simulink library "halin"  (R2021b)
settings: Solver=VariableStepAuto  StartTime=0.0  StopTime=10.0  RelTol=1e-3
undefined symbols (not defined in the file): TRUE
libraries: FVT_lib x37, hcu_lib x31
(part 2 of 4)

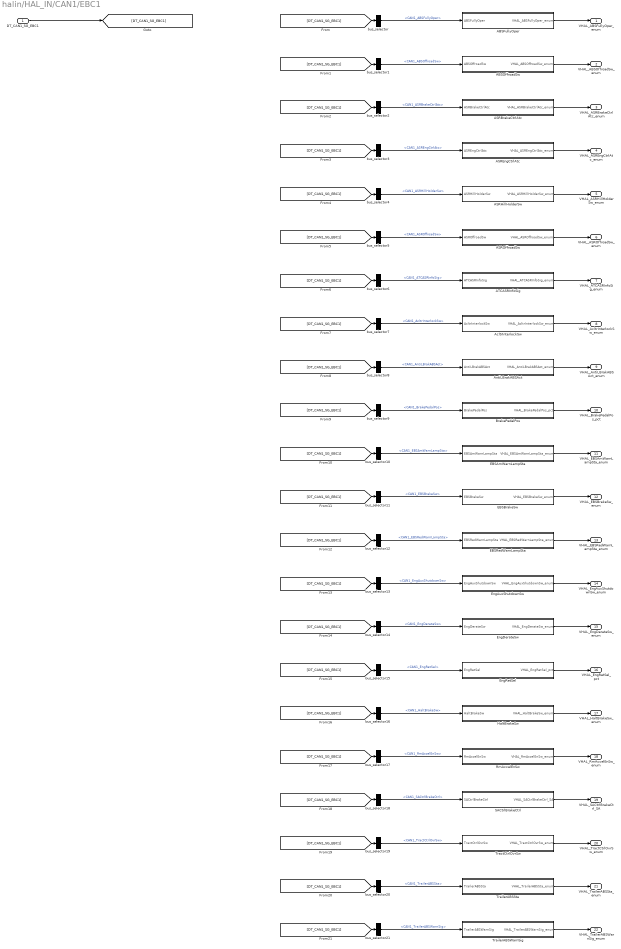
== system halin/HAL_IN/CAN1/EBC1 ==
  DT_CAN1_SG_EBC1 : Inport
  ABSFullyOper : Subsystem
  ABSOffroadSw : Subsystem
  ASRBrakeCtrlAtc : Subsystem
  ASREngCtrlAtc : Subsystem
  ASRHillHolderSw : Subsystem
  ASROffroadSw : Subsystem
  ATCASRInfoSig : Subsystem
  AcltrInterlockSw : Subsystem
  AntiLBrakABSAct : Subsystem
  BrakePedalPos : Subsystem
  EBSAmWarnLampSta : Subsystem
  EBSBrakeSw : Subsystem
  EBSRedWarnLampSta : Subsystem
  EngAuxShutdownSw : Subsystem
  EngDerateSw : Subsystem
  EngRetSel : Subsystem
  HaltBrakeSw : Subsystem
  RmAccelEnSw : Subsystem
  SACtrlBrakeCtrl : Subsystem
  TractCtrlOvrSw : Subsystem
  TrailerABSSta : Subsystem
  TrailerABSWarnSig : Subsystem
  bus_selector : BusSelector  OutputSignals=CAN1_ABSFullyOper
  bus_selector1 : BusSelector  OutputSignals=CAN1_ABSOffroadSw
  bus_selector10 : BusSelector  OutputSignals=CAN1_EBSAmWarnLampSta
  bus_selector11 : BusSelector  OutputSignals=CAN1_EBSBrakeSw
  bus_selector12 : BusSelector  OutputSignals=CAN1_EBSRedWarnLampSta
  bus_selector13 : BusSelector  OutputSignals=CAN1_EngAuxShutdownSw
  bus_selector14 : BusSelector  OutputSignals=CAN1_EngDerateSw
  bus_selector15 : BusSelector  OutputSignals=CAN1_EngRetSel
  bus_selector16 : BusSelector  OutputSignals=CAN1_HaltBrakeSw
  bus_selector17 : BusSelector  OutputSignals=CAN1_RmAccelEnSw
  bus_selector18 : BusSelector  OutputSignals=CAN1_SACtrlBrakeCtrl
  bus_selector19 : BusSelector  OutputSignals=CAN1_TractCtrlOvrSw
  bus_selector2 : BusSelector  OutputSignals=CAN1_ASRBrakeCtrlAtc
  bus_selector20 : BusSelector  OutputSignals=CAN1_TrailerABSSta
  bus_selector21 : BusSelector  OutputSignals=CAN1_TrailerABSWarnSig
  bus_selector3 : BusSelector  OutputSignals=CAN1_ASREngCtrlAtc
  bus_selector4 : BusSelector  OutputSignals=CAN1_ASRHillHolderSw
  bus_selector5 : BusSelector  OutputSignals=CAN1_ASROffroadSw
  bus_selector6 : BusSelector  OutputSignals=CAN1_ATCASRInfoSig
  bus_selector7 : BusSelector  OutputSignals=CAN1_AcltrInterlockSw
  bus_selector8 : BusSelector  OutputSignals=CAN1_AntiLBrakABSAct
  bus_selector9 : BusSelector  OutputSignals=CAN1_BrakePedalPos
  VHAL_ABSFullyOper_enum : Outport
  VHAL_ABSOffroadSw_enum : Outport  Port=2
  VHAL_ASRBrakeCtrlAtc_enum : Outport  Port=3
  VHAL_ASREngCtrlAtc_enum : Outport  Port=4
  VHAL_ASRHillHolderSw_enum : Outport  Port=5
  VHAL_ASROffroadSw_enum : Outport  Port=6
  VHAL_ATCASRInfoSig_enum : Outport  Port=7
  VHAL_AcltrInterlockSw_enum : Outport  Port=8
  VHAL_AntiLBrakABSAct_enum : Outport  Port=9
  VHAL_BrakePedalPos_pct : Outport  Port=10
  VHAL_EBSAmWarnLampSta_enum : Outport  Port=11
  VHAL_EBSBrakeSw_enum : Outport  Port=12
  VHAL_EBSRedWarnLampSta_enum : Outport  Port=13
  VHAL_EngAuxShutdownSw_enum : Outport  Port=14
  VHAL_EngDerateSw_enum : Outport  Port=15
  VHAL_EngRetSel_pct : Outport  Port=16
  VHAL_HaltBrakeSw_enum : Outport  Port=17
  VHAL_RmAccelEnSw_enum : Outport  Port=18
  VHAL_SACtrlBrakeCtrl_SA : Outport  Port=19
  VHAL_TractCtrlOvrSw_enum : Outport  Port=20
  VHAL_TrailerABSSta_enum : Outport  Port=21
  VHAL_TrailerABSWarnSig_enum : Outport  Port=22
  wires:
  DT_CAN1_SG_EBC1/1 -> [DT_CAN1_SG_EBC1]
  [DT_CAN1_SG_EBC1] -> bus_selector/1
  bus_selector/1 -> ABSFullyOper/1(ABSFullyOper)  "<CAN1_ABSFullyOper>"
  ABSFullyOper/1(VHAL_ABSFullyOper_enum) -> VHAL_ABSFullyOper_enum/1
  [DT_CAN1_SG_EBC1] -> bus_selector1/1
  bus_selector1/1 -> ABSOffroadSw/1(ABSOffroadSw)  "<CAN1_ABSOffroadSw>"
  ABSOffroadSw/1(VHAL_ABSOffroadSw_enum) -> VHAL_ABSOffroadSw_enum/1
  [DT_CAN1_SG_EBC1] -> bus_selector2/1
  bus_selector2/1 -> ASRBrakeCtrlAtc/1(ASRBrakeCtrlAtc)  "<CAN1_ASRBrakeCtrlAtc>"
  ASRBrakeCtrlAtc/1(VHAL_ASRBrakeCtrlAtc_enum) -> VHAL_ASRBrakeCtrlAtc_enum/1
  [DT_CAN1_SG_EBC1] -> bus_selector3/1
  bus_selector3/1 -> ASREngCtrlAtc/1(ASREngCtrlAtc)  "<CAN1_ASREngCtrlAtc>"
  ASREngCtrlAtc/1(VHAL_ASREngCtrlAtc_enum) -> VHAL_ASREngCtrlAtc_enum/1
  [DT_CAN1_SG_EBC1] -> bus_selector4/1
  bus_selector4/1 -> ASRHillHolderSw/1(ASRHillHolderSw)  "<CAN1_ASRHillHolderSw>"
  ASRHillHolderSw/1(VHAL_ASRHillHolderSw_enum) -> VHAL_ASRHillHolderSw_enum/1
  [DT_CAN1_SG_EBC1] -> bus_selector5/1
  bus_selector5/1 -> ASROffroadSw/1(ASROffroadSw)  "<CAN1_ASROffroadSw>"
  ASROffroadSw/1(VHAL_ASROffroadSw_enum) -> VHAL_ASROffroadSw_enum/1
  [DT_CAN1_SG_EBC1] -> bus_selector6/1
  bus_selector6/1 -> ATCASRInfoSig/1(ATCASRInfoSig)  "<CAN1_ATCASRInfoSig>"
  ATCASRInfoSig/1(VHAL_ATCASRInfoSig_enum) -> VHAL_ATCASRInfoSig_enum/1
  [DT_CAN1_SG_EBC1] -> bus_selector7/1
  bus_selector7/1 -> AcltrInterlockSw/1(AcltrInterlockSw)  "<CAN1_AcltrInterlockSw>"
  AcltrInterlockSw/1(VHAL_AcltrInterlockSw_enum) -> VHAL_AcltrInterlockSw_enum/1
  [DT_CAN1_SG_EBC1] -> bus_selector8/1
  bus_selector8/1 -> AntiLBrakABSAct/1(AntiLBrakABSAct)  "<CAN1_AntiLBrakABSAct>"
  AntiLBrakABSAct/1(VHAL_AntiLBrakABSAct_enum) -> VHAL_AntiLBrakABSAct_enum/1
  [DT_CAN1_SG_EBC1] -> bus_selector9/1
  bus_selector9/1 -> BrakePedalPos/1(BrakePedalPos)  "<CAN1_BrakePedalPos>"
  BrakePedalPos/1(VHAL_BrakePedalPos_pct) -> VHAL_BrakePedalPos_pct/1
  [DT_CAN1_SG_EBC1] -> bus_selector10/1
  bus_selector10/1 -> EBSAmWarnLampSta/1(EBSAmWarnLampSta)  "<CAN1_EBSAmWarnLampSta>"
  EBSAmWarnLampSta/1(VHAL_EBSAmWarnLampSta_enum) -> VHAL_EBSAmWarnLampSta_enum/1
  [DT_CAN1_SG_EBC1] -> bus_selector11/1
  bus_selector11/1 -> EBSBrakeSw/1(EBSBrakeSw)  "<CAN1_EBSBrakeSw>"
  EBSBrakeSw/1(VHAL_EBSBrakeSw_enum) -> VHAL_EBSBrakeSw_enum/1
  [DT_CAN1_SG_EBC1] -> bus_selector12/1
  bus_selector12/1 -> EBSRedWarnLampSta/1(EBSRedWarnLampSta)  "<CAN1_EBSRedWarnLampSta>"
  EBSRedWarnLampSta/1(VHAL_EBSRedWarnLampSta_enum) -> VHAL_EBSRedWarnLampSta_enum/1
  [DT_CAN1_SG_EBC1] -> bus_selector13/1
  bus_selector13/1 -> EngAuxShutdownSw/1(EngAuxShutdownSw)  "<CAN1_EngAuxShutdownSw>"
  EngAuxShutdownSw/1(VHAL_EngAuxShutdownSw_enum) -> VHAL_EngAuxShutdownSw_enum/1
  [DT_CAN1_SG_EBC1] -> bus_selector14/1
  bus_selector14/1 -> EngDerateSw/1(EngDerateSw)  "<CAN1_EngDerateSw>"
  EngDerateSw/1(VHAL_EngDerateSw_enum) -> VHAL_EngDerateSw_enum/1
  [DT_CAN1_SG_EBC1] -> bus_selector15/1
  bus_selector15/1 -> EngRetSel/1(EngRetSel)  "<CAN1_EngRetSel>"
  EngRetSel/1(VHAL_EngRetSel_pct) -> VHAL_EngRetSel_pct/1
  [DT_CAN1_SG_EBC1] -> bus_selector16/1
  bus_selector16/1 -> HaltBrakeSw/1(HaltBrakeSw)  "<CAN1_HaltBrakeSw>"
  HaltBrakeSw/1(VHAL_HaltBrakeSw_enum) -> VHAL_HaltBrakeSw_enum/1
  [DT_CAN1_SG_EBC1] -> bus_selector17/1
  bus_selector17/1 -> RmAccelEnSw/1(RmAccelEnSw)  "<CAN1_RmAccelEnSw>"
  RmAccelEnSw/1(VHAL_RmAccelEnSw_enum) -> VHAL_RmAccelEnSw_enum/1
  [DT_CAN1_SG_EBC1] -> bus_selector18/1
  bus_selector18/1 -> SACtrlBrakeCtrl/1(SACtrlBrakeCtrl)  "<CAN1_SACtrlBrakeCtrl>"
  SACtrlBrakeCtrl/1(VHAL_SACtrlBrakeCtrl_SA) -> VHAL_SACtrlBrakeCtrl_SA/1
  [DT_CAN1_SG_EBC1] -> bus_selector19/1
  bus_selector19/1 -> TractCtrlOvrSw/1(TractCtrlOvrSw)  "<CAN1_TractCtrlOvrSw>"
  TractCtrlOvrSw/1(VHAL_TractCtrlOvrSw_enum) -> VHAL_TractCtrlOvrSw_enum/1
  [DT_CAN1_SG_EBC1] -> bus_selector20/1
  bus_selector20/1 -> TrailerABSSta/1(TrailerABSSta)  "<CAN1_TrailerABSSta>"
  TrailerABSSta/1(VHAL_TrailerABSSta_enum) -> VHAL_TrailerABSSta_enum/1
  [DT_CAN1_SG_EBC1] -> bus_selector21/1
  bus_selector21/1 -> TrailerABSWarnSig/1(TrailerABSWarnSig)  "<CAN1_TrailerABSWarnSig>"
  TrailerABSWarnSig/1(VHAL_TrailerABSWarnSig_enum) -> VHAL_TrailerABSWarnSig_enum/1

== system halin/HAL_IN/CAN1/EBC2 ==
  DT_CAN1_SG_EBC2 : Inport
  FASpeed : Subsystem
  RelaSpdFALWheel : Subsystem
  RelaSpdFARWheel : Subsystem
  bus_selector : BusSelector  OutputSignals=CAN1_FASpeed
  bus_selector1 : BusSelector  OutputSignals=CAN1_RelaSpdFALWheel
  bus_selector2 : BusSelector  OutputSignals=CAN1_RelaSpdFARWheel
  VHAL_FASpeed_kph : Outport
  VHAL_RelaSpdFALWheel_kph : Outport  Port=2
  VHAL_RelaSpdFARWheel_kph : Outport  Port=3
  wires:
  DT_CAN1_SG_EBC2/1 -> [DT_CAN1_SG_EBC2]
  [DT_CAN1_SG_EBC2] -> bus_selector/1
  bus_selector/1 -> FASpeed/1(FASpeed)  "<CAN1_FASpeed>"
  FASpeed/1(VHAL_FASpeed_kph) -> VHAL_FASpeed_kph/1
  [DT_CAN1_SG_EBC2] -> bus_selector1/1
  bus_selector1/1 -> RelaSpdFALWheel/1(RelaSpdFALWheel)  "<CAN1_RelaSpdFALWheel>"
  RelaSpdFALWheel/1(VHAL_RelaSpdFALWheel_kph) -> VHAL_RelaSpdFALWheel_kph/1
  [DT_CAN1_SG_EBC2] -> bus_selector2/1
  bus_selector2/1 -> RelaSpdFARWheel/1(RelaSpdFARWheel)  "<CAN1_RelaSpdFARWheel>"
  RelaSpdFARWheel/1(VHAL_RelaSpdFARWheel_kph) -> VHAL_RelaSpdFARWheel_kph/1

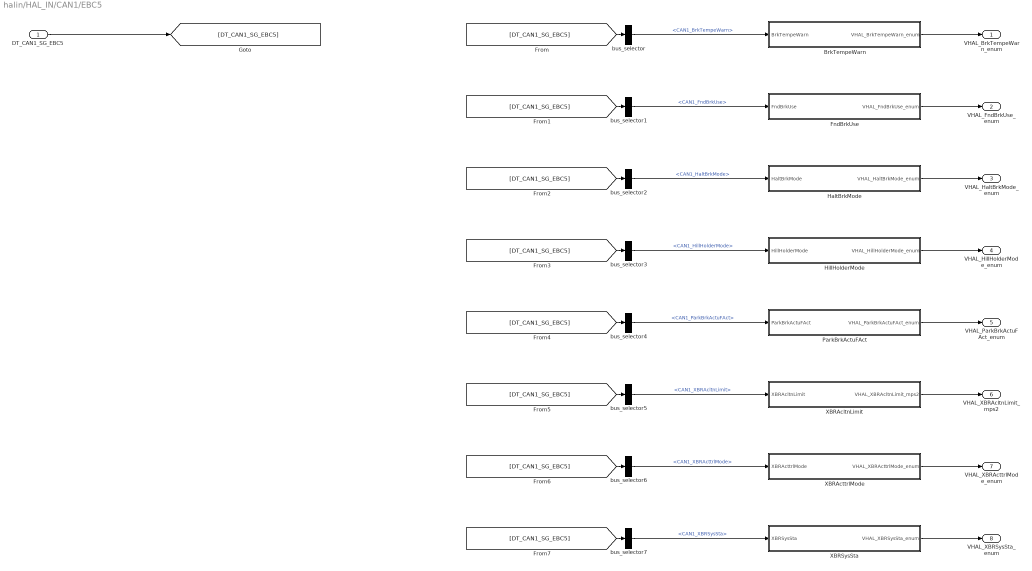
== system halin/HAL_IN/CAN1/EBC5 ==
  DT_CAN1_SG_EBC5 : Inport
  BrkTempeWarn : Subsystem
  FndBrkUse : Subsystem
  HaltBrkMode : Subsystem
  HillHolderMode : Subsystem
  ParkBrkActuFAct : Subsystem
  XBRAcltnLimit : Subsystem
  XBRActtrlMode : Subsystem
  XBRSysSta : Subsystem
  bus_selector : BusSelector  OutputSignals=CAN1_BrkTempeWarn
  bus_selector1 : BusSelector  OutputSignals=CAN1_FndBrkUse
  bus_selector2 : BusSelector  OutputSignals=CAN1_HaltBrkMode
  bus_selector3 : BusSelector  OutputSignals=CAN1_HillHolderMode
  bus_selector4 : BusSelector  OutputSignals=CAN1_ParkBrkActuFAct
  bus_selector5 : BusSelector  OutputSignals=CAN1_XBRAcltnLimit
  bus_selector6 : BusSelector  OutputSignals=CAN1_XBRActtrlMode
  bus_selector7 : BusSelector  OutputSignals=CAN1_XBRSysSta
  VHAL_BrkTempeWarn_enum : Outport
  VHAL_FndBrkUse_enum : Outport  Port=2
  VHAL_HaltBrkMode_enum : Outport  Port=3
  VHAL_HillHolderMode_enum : Outport  Port=4
  VHAL_ParkBrkActuFAct_enum : Outport  Port=5
  VHAL_XBRAcltnLimit_mps2 : Outport  Port=6
  VHAL_XBRActtrlMode_enum : Outport  Port=7
  VHAL_XBRSysSta_enum : Outport  Port=8
  wires:
  DT_CAN1_SG_EBC5/1 -> [DT_CAN1_SG_EBC5]
  [DT_CAN1_SG_EBC5] -> bus_selector/1
  bus_selector/1 -> BrkTempeWarn/1(BrkTempeWarn)  "<CAN1_BrkTempeWarn>"
  BrkTempeWarn/1(VHAL_BrkTempeWarn_enum) -> VHAL_BrkTempeWarn_enum/1
  [DT_CAN1_SG_EBC5] -> bus_selector1/1
  bus_selector1/1 -> FndBrkUse/1(FndBrkUse)  "<CAN1_FndBrkUse>"
  FndBrkUse/1(VHAL_FndBrkUse_enum) -> VHAL_FndBrkUse_enum/1
  [DT_CAN1_SG_EBC5] -> bus_selector2/1
  bus_selector2/1 -> HaltBrkMode/1(HaltBrkMode)  "<CAN1_HaltBrkMode>"
  HaltBrkMode/1(VHAL_HaltBrkMode_enum) -> VHAL_HaltBrkMode_enum/1
  [DT_CAN1_SG_EBC5] -> bus_selector3/1
  bus_selector3/1 -> HillHolderMode/1(HillHolderMode)  "<CAN1_HillHolderMode>"
  HillHolderMode/1(VHAL_HillHolderMode_enum) -> VHAL_HillHolderMode_enum/1
  [DT_CAN1_SG_EBC5] -> bus_selector4/1
  bus_selector4/1 -> ParkBrkActuFAct/1(ParkBrkActuFAct)  "<CAN1_ParkBrkActuFAct>"
  ParkBrkActuFAct/1(VHAL_ParkBrkActuFAct_enum) -> VHAL_ParkBrkActuFAct_enum/1
  [DT_CAN1_SG_EBC5] -> bus_selector5/1
  bus_selector5/1 -> XBRAcltnLimit/1(XBRAcltnLimit)  "<CAN1_XBRAcltnLimit>"
  XBRAcltnLimit/1(VHAL_XBRAcltnLimit_mps2) -> VHAL_XBRAcltnLimit_mps2/1
  [DT_CAN1_SG_EBC5] -> bus_selector6/1
  bus_selector6/1 -> XBRActtrlMode/1(XBRActtrlMode)  "<CAN1_XBRActtrlMode>"
  XBRActtrlMode/1(VHAL_XBRActtrlMode_enum) -> VHAL_XBRActtrlMode_enum/1
  [DT_CAN1_SG_EBC5] -> bus_selector7/1
  bus_selector7/1 -> XBRSysSta/1(XBRSysSta)  "<CAN1_XBRSysSta>"
  XBRSysSta/1(VHAL_XBRSysSta_enum) -> VHAL_XBRSysSta_enum/1

== system halin/HAL_IN/CAN1/ECAS_DM1 ==
  DT_CAN1_SG_ECAS_DM1 : Inport
  ECASAWarmLampSta : Subsystem
  bus_selector : BusSelector  OutputSignals=CAN1_ECASAWarmLampSta
  VHAL_ECASAWarmLampSta_enum : Outport
  wires:
  DT_CAN1_SG_ECAS_DM1/1 -> [DT_CAN1_SG_ECAS_DM1]
  [DT_CAN1_SG_ECAS_DM1] -> bus_selector/1
  bus_selector/1 -> ECASAWarmLampSta/1(ECASAWarmLampSta)  "<CAN1_ECASAWarmLampSta>"
  ECASAWarmLampSta/1(VHAL_ECASAWarmLampSta_enum) -> VHAL_ECASAWarmLampSta_enum/1

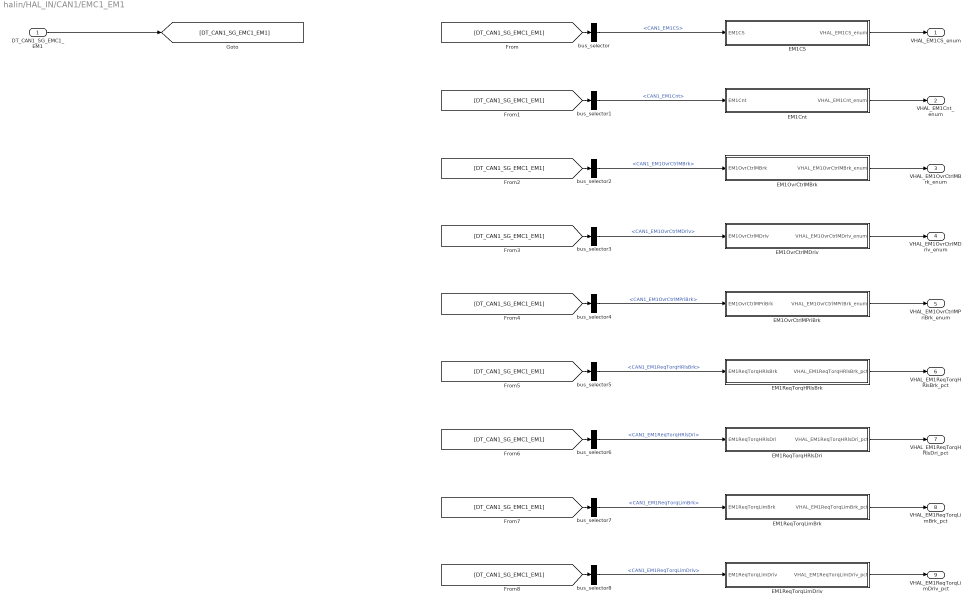
== system halin/HAL_IN/CAN1/EMC1_EM1 ==
  DT_CAN1_SG_EMC1_EM1 : Inport
  EM1CS : Subsystem
  EM1Cnt : Subsystem
  EM1OvrCtrlMBrk : Subsystem
  EM1OvrCtrlMDriv : Subsystem
  EM1OvrCtrlMPriBrk : Subsystem
  EM1ReqTorqHRlsBrk : Subsystem
  EM1ReqTorqHRlsDri : Subsystem
  EM1ReqTorqLimBrk : Subsystem
  EM1ReqTorqLimDriv : Subsystem
  bus_selector : BusSelector  OutputSignals=CAN1_EM1CS
  bus_selector1 : BusSelector  OutputSignals=CAN1_EM1Cnt
  bus_selector2 : BusSelector  OutputSignals=CAN1_EM1OvrCtrlMBrk
  bus_selector3 : BusSelector  OutputSignals=CAN1_EM1OvrCtrlMDriv
  bus_selector4 : BusSelector  OutputSignals=CAN1_EM1OvrCtrlMPriBrk
  bus_selector5 : BusSelector  OutputSignals=CAN1_EM1ReqTorqHRlsBrk
  bus_selector6 : BusSelector  OutputSignals=CAN1_EM1ReqTorqHRlsDri
  bus_selector7 : BusSelector  OutputSignals=CAN1_EM1ReqTorqLimBrk
  bus_selector8 : BusSelector  OutputSignals=CAN1_EM1ReqTorqLimDriv
  VHAL_EM1CS_enum : Outport
  VHAL_EM1Cnt_enum : Outport  Port=2
  VHAL_EM1OvrCtrlMBrk_enum : Outport  Port=3
  VHAL_EM1OvrCtrlMDriv_enum : Outport  Port=4
  VHAL_EM1OvrCtrlMPriBrk_enum : Outport  Port=5
  VHAL_EM1ReqTorqHRlsBrk_pct : Outport  Port=6
  VHAL_EM1ReqTorqHRlsDri_pct : Outport  Port=7
  VHAL_EM1ReqTorqLimBrk_pct : Outport  Port=8
  VHAL_EM1ReqTorqLimDriv_pct : Outport  Port=9
  wires:
  DT_CAN1_SG_EMC1_EM1/1 -> [DT_CAN1_SG_EMC1_EM1]
  [DT_CAN1_SG_EMC1_EM1] -> bus_selector/1
  bus_selector/1 -> EM1CS/1(EM1CS)  "<CAN1_EM1CS>"
  EM1CS/1(VHAL_EM1CS_enum) -> VHAL_EM1CS_enum/1
  [DT_CAN1_SG_EMC1_EM1] -> bus_selector1/1
  bus_selector1/1 -> EM1Cnt/1(EM1Cnt)  "<CAN1_EM1Cnt>"
  EM1Cnt/1(VHAL_EM1Cnt_enum) -> VHAL_EM1Cnt_enum/1
  [DT_CAN1_SG_EMC1_EM1] -> bus_selector2/1
  bus_selector2/1 -> EM1OvrCtrlMBrk/1(EM1OvrCtrlMBrk)  "<CAN1_EM1OvrCtrlMBrk>"
  EM1OvrCtrlMBrk/1(VHAL_EM1OvrCtrlMBrk_enum) -> VHAL_EM1OvrCtrlMBrk_enum/1
  [DT_CAN1_SG_EMC1_EM1] -> bus_selector3/1
  bus_selector3/1 -> EM1OvrCtrlMDriv/1(EM1OvrCtrlMDriv)  "<CAN1_EM1OvrCtrlMDriv>"
  EM1OvrCtrlMDriv/1(VHAL_EM1OvrCtrlMDriv_enum) -> VHAL_EM1OvrCtrlMDriv_enum/1
  [DT_CAN1_SG_EMC1_EM1] -> bus_selector4/1
  bus_selector4/1 -> EM1OvrCtrlMPriBrk/1(EM1OvrCtrlMPriBrk)  "<CAN1_EM1OvrCtrlMPriBrk>"
  EM1OvrCtrlMPriBrk/1(VHAL_EM1OvrCtrlMPriBrk_enum) -> VHAL_EM1OvrCtrlMPriBrk_enum/1
  [DT_CAN1_SG_EMC1_EM1] -> bus_selector5/1
  bus_selector5/1 -> EM1ReqTorqHRlsBrk/1(EM1ReqTorqHRlsBrk)  "<CAN1_EM1ReqTorqHRlsBrk>"
  EM1ReqTorqHRlsBrk/1(VHAL_EM1ReqTorqHRlsBrk_pct) -> VHAL_EM1ReqTorqHRlsBrk_pct/1
  [DT_CAN1_SG_EMC1_EM1] -> bus_selector6/1
  bus_selector6/1 -> EM1ReqTorqHRlsDri/1(EM1ReqTorqHRlsDri)  "<CAN1_EM1ReqTorqHRlsDri>"
  EM1ReqTorqHRlsDri/1(VHAL_EM1ReqTorqHRlsDri_pct) -> VHAL_EM1ReqTorqHRlsDri_pct/1
  [DT_CAN1_SG_EMC1_EM1] -> bus_selector7/1
  bus_selector7/1 -> EM1ReqTorqLimBrk/1(EM1ReqTorqLimBrk)  "<CAN1_EM1ReqTorqLimBrk>"
  EM1ReqTorqLimBrk/1(VHAL_EM1ReqTorqLimBrk_pct) -> VHAL_EM1ReqTorqLimBrk_pct/1
  [DT_CAN1_SG_EMC1_EM1] -> bus_selector8/1
  bus_selector8/1 -> EM1ReqTorqLimDriv/1(EM1ReqTorqLimDriv)  "<CAN1_EM1ReqTorqLimDriv>"
  EM1ReqTorqLimDriv/1(VHAL_EM1ReqTorqLimDriv_pct) -> VHAL_EM1ReqTorqLimDriv_pct/1

== system halin/HAL_IN/CAN1/HRW ==
  DT_CAN1_SG_HRW : Inport
  WhlSpeedFL : Subsystem
  bus_selector : BusSelector  OutputSignals=CAN1_WhlSpeed_FL
  VHAL_WhlSpeedFL_kph : Outport
  wires:
  DT_CAN1_SG_HRW/1 -> [DT_CAN1_SG_HRW]
  [DT_CAN1_SG_HRW] -> bus_selector/1
  bus_selector/1 -> WhlSpeedFL/1(WhlSpeed_FL)  "<CAN1_WhlSpeed_FL>"
  WhlSpeedFL/1(VHAL_WhlSpeedFL_kph) -> VHAL_WhlSpeedFL_kph/1

== system halin/HAL_IN/CAN1/TC1 ==
  DT_CAN1_SG_TC1 : Inport
  DrivDirF : Subsystem
  TransReqGear : Subsystem
  bus_selector : BusSelector  OutputSignals=CAN1_DrivDirF
  bus_selector1 : BusSelector  OutputSignals=CAN1_TransReqGear
  VHAL_DrivDirF_enum : Outport
  VHAL_TransReqGear_enum : Outport  Port=2
  wires:
  DT_CAN1_SG_TC1/1 -> [DT_CAN1_SG_TC1]
  [DT_CAN1_SG_TC1] -> bus_selector/1
  bus_selector/1 -> DrivDirF/1(DrivDirF)  "<CAN1_DrivDirF>"
  DrivDirF/1(VHAL_DrivDirF_enum) -> VHAL_DrivDirF_enum/1
  [DT_CAN1_SG_TC1] -> bus_selector1/1
  bus_selector1/1 -> TransReqGear/1(TransReqGear)  "<CAN1_TransReqGear>"
  TransReqGear/1(VHAL_TransReqGear_enum) -> VHAL_TransReqGear_enum/1

== system halin/HAL_IN/CAN1/VHAL_CANMsgInvalidACBTMSC10000_flg ==
  Cast To Boolean13 : DataTypeConversion  OutDataTypeStr=boolean
  Constant : Constant  Value=TRUE
  Latch13 : hcu_lib/Basic_Blocks/Latch
  Switch13 : Switch  Criteria=u2 ~= 0
  Unit Delay : UnitDelay  SampleTime=-1  HasFrameUpgradeWarning=on
  UnitConverter : DataTypeConversion  OutDataTypeStr=boolean
  Out : Outport
  wires:
  Constant/1 -> Switch13/3
  Unit Delay/1 -> Cast To Boolean13/1
  Cast To Boolean13/1 -> Switch13/1, Latch13/1
  Switch13/1 -> UnitConverter/1
  Latch13/1 -> Switch13/2
  UnitConverter/1 -> Unit Delay/1, Out/1  "VHAL_CANMsgInvalidACBTMSC10000_flg"

== system halin/HAL_IN/CAN1/VHAL_CANMsgInvalidACBTMSC10001_flg ==
  Cast To Boolean13 : DataTypeConversion  OutDataTypeStr=boolean
  Constant : Constant  Value=TRUE
  Latch13 : hcu_lib/Basic_Blocks/Latch
  Switch13 : Switch  Criteria=u2 ~= 0
  Unit Delay : UnitDelay  SampleTime=-1  HasFrameUpgradeWarning=on
  UnitConverter : DataTypeConversion  OutDataTypeStr=boolean
  Out : Outport
  wires:
  Constant/1 -> Switch13/3
  Unit Delay/1 -> Cast To Boolean13/1
  Cast To Boolean13/1 -> Switch13/1, Latch13/1
  Switch13/1 -> UnitConverter/1
  Latch13/1 -> Switch13/2
  UnitConverter/1 -> Unit Delay/1, Out/1  "VHAL_CANMsgInvalidACBTMSC10001_flg"

== system halin/HAL_IN/CAN1/VHAL_CANMsgInvalidACBTMSC10004_flg ==
  Cast To Boolean13 : DataTypeConversion  OutDataTypeStr=boolean
  Constant : Constant  Value=TRUE
  Latch13 : hcu_lib/Basic_Blocks/Latch
  Switch13 : Switch  Criteria=u2 ~= 0
  Unit Delay : UnitDelay  SampleTime=-1  HasFrameUpgradeWarning=on
  UnitConverter : DataTypeConversion  OutDataTypeStr=boolean
  Out : Outport
  wires:
  Constant/1 -> Switch13/3
  Unit Delay/1 -> Cast To Boolean13/1
  Cast To Boolean13/1 -> Switch13/1, Latch13/1
  Switch13/1 -> UnitConverter/1
  Latch13/1 -> Switch13/2
  UnitConverter/1 -> Unit Delay/1, Out/1  "VHAL_CANMsgInvalidACBTMSC10004_flg"

== system halin/HAL_IN/CAN1/VHAL_CANMsgInvalidACBTMSC50000_flg ==
  Cast To Boolean13 : DataTypeConversion  OutDataTypeStr=boolean
  Constant : Constant  Value=TRUE
  Latch13 : hcu_lib/Basic_Blocks/Latch
  Switch13 : Switch  Criteria=u2 ~= 0
  Unit Delay : UnitDelay  SampleTime=-1  HasFrameUpgradeWarning=on
  UnitConverter : DataTypeConversion  OutDataTypeStr=boolean
  Out : Outport
  wires:
  Constant/1 -> Switch13/3
  Unit Delay/1 -> Cast To Boolean13/1
  Cast To Boolean13/1 -> Switch13/1, Latch13/1
  Switch13/1 -> UnitConverter/1
  Latch13/1 -> Switch13/2
  UnitConverter/1 -> Unit Delay/1, Out/1  "VHAL_CANMsgInvalidACBTMSC50000_flg"

== system halin/HAL_IN/CAN1/VHAL_CANMsgInvalidASC1A_flg ==
  Cast To Boolean13 : DataTypeConversion  OutDataTypeStr=boolean
  Constant : Constant  Value=TRUE
  Latch13 : hcu_lib/Basic_Blocks/Latch
  Switch13 : Switch  Criteria=u2 ~= 0
  Unit Delay : UnitDelay  SampleTime=-1  HasFrameUpgradeWarning=on
  UnitConverter : DataTypeConversion  OutDataTypeStr=boolean
  Out : Outport
  wires:
  Constant/1 -> Switch13/3
  Unit Delay/1 -> Cast To Boolean13/1
  Cast To Boolean13/1 -> Switch13/1, Latch13/1
  Switch13/1 -> UnitConverter/1
  Latch13/1 -> Switch13/2
  UnitConverter/1 -> Unit Delay/1, Out/1  "VHAL_CANMsgInvalidASC1A_flg"

== system halin/HAL_IN/CAN1/VHAL_CANMsgInvalidEBC1_flg ==
  Cast To Boolean13 : DataTypeConversion  OutDataTypeStr=boolean
  Constant : Constant  Value=TRUE
  Latch13 : hcu_lib/Basic_Blocks/Latch
  Switch13 : Switch  Criteria=u2 ~= 0
  Unit Delay : UnitDelay  SampleTime=-1  HasFrameUpgradeWarning=on
  UnitConverter : DataTypeConversion  OutDataTypeStr=boolean
  Out : Outport
  wires:
  Constant/1 -> Switch13/3
  Unit Delay/1 -> Cast To Boolean13/1
  Cast To Boolean13/1 -> Switch13/1, Latch13/1
  Switch13/1 -> UnitConverter/1
  Latch13/1 -> Switch13/2
  UnitConverter/1 -> Unit Delay/1, Out/1  "VHAL_CANMsgInvalidEBC1_flg"

== system halin/HAL_IN/CAN1/VHAL_CANMsgInvalidEBC2_flg ==
  Cast To Boolean13 : DataTypeConversion  OutDataTypeStr=boolean
  Constant : Constant  Value=TRUE
  Latch13 : hcu_lib/Basic_Blocks/Latch
  Switch13 : Switch  Criteria=u2 ~= 0
  Unit Delay : UnitDelay  SampleTime=-1  HasFrameUpgradeWarning=on
  UnitConverter : DataTypeConversion  OutDataTypeStr=boolean
  Out : Outport
  wires:
  Constant/1 -> Switch13/3
  Unit Delay/1 -> Cast To Boolean13/1
  Cast To Boolean13/1 -> Switch13/1, Latch13/1
  Switch13/1 -> UnitConverter/1
  Latch13/1 -> Switch13/2
  UnitConverter/1 -> Unit Delay/1, Out/1  "VHAL_CANMsgInvalidEBC2_flg"

== system halin/HAL_IN/CAN1/VHAL_CANMsgInvalidEBC5_flg ==
  Cast To Boolean13 : DataTypeConversion  OutDataTypeStr=boolean
  Constant : Constant  Value=TRUE
  Latch13 : hcu_lib/Basic_Blocks/Latch
  Switch13 : Switch  Criteria=u2 ~= 0
  Unit Delay : UnitDelay  SampleTime=-1  HasFrameUpgradeWarning=on
  UnitConverter : DataTypeConversion  OutDataTypeStr=boolean
  Out : Outport
  wires:
  Constant/1 -> Switch13/3
  Unit Delay/1 -> Cast To Boolean13/1
  Cast To Boolean13/1 -> Switch13/1, Latch13/1
  Switch13/1 -> UnitConverter/1
  Latch13/1 -> Switch13/2
  UnitConverter/1 -> Unit Delay/1, Out/1  "VHAL_CANMsgInvalidEBC5_flg"

== system halin/HAL_IN/CAN1/VHAL_CANMsgInvalidECASDM1_flg ==
  Cast To Boolean13 : DataTypeConversion  OutDataTypeStr=boolean
  Constant : Constant  Value=TRUE
  Latch13 : hcu_lib/Basic_Blocks/Latch
  Switch13 : Switch  Criteria=u2 ~= 0
  Unit Delay : UnitDelay  SampleTime=-1  HasFrameUpgradeWarning=on
  UnitConverter : DataTypeConversion  OutDataTypeStr=boolean
  Out : Outport
  wires:
  Constant/1 -> Switch13/3
  Unit Delay/1 -> Cast To Boolean13/1
  Cast To Boolean13/1 -> Switch13/1, Latch13/1
  Switch13/1 -> UnitConverter/1
  Latch13/1 -> Switch13/2
  UnitConverter/1 -> Unit Delay/1, Out/1  "VHAL_CANMsgInvalidECASDM1_flg"

== system halin/HAL_IN/CAN1/VHAL_CANMsgInvalidEMC1EM1_flg ==
  Cast To Boolean13 : DataTypeConversion  OutDataTypeStr=boolean
  Constant : Constant  Value=TRUE
  Latch13 : hcu_lib/Basic_Blocks/Latch
  Switch13 : Switch  Criteria=u2 ~= 0
  Unit Delay : UnitDelay  SampleTime=-1  HasFrameUpgradeWarning=on
  UnitConverter : DataTypeConversion  OutDataTypeStr=boolean
  Out : Outport
  wires:
  Constant/1 -> Switch13/3
  Unit Delay/1 -> Cast To Boolean13/1
  Cast To Boolean13/1 -> Switch13/1, Latch13/1
  Switch13/1 -> UnitConverter/1
  Latch13/1 -> Switch13/2
  UnitConverter/1 -> Unit Delay/1, Out/1  "VHAL_CANMsgInvalidEMC1EM1_flg"

== system halin/HAL_IN/CAN1/VHAL_CANMsgInvalidHRW_flg ==
  Cast To Boolean13 : DataTypeConversion  OutDataTypeStr=boolean
  Constant : Constant  Value=TRUE
  Latch13 : hcu_lib/Basic_Blocks/Latch
  Switch13 : Switch  Criteria=u2 ~= 0
  Unit Delay : UnitDelay  SampleTime=-1  HasFrameUpgradeWarning=on
  UnitConverter : DataTypeConversion  OutDataTypeStr=boolean
  Out : Outport
  wires:
  Constant/1 -> Switch13/3
  Unit Delay/1 -> Cast To Boolean13/1
  Cast To Boolean13/1 -> Switch13/1, Latch13/1
  Switch13/1 -> UnitConverter/1
  Latch13/1 -> Switch13/2
  UnitConverter/1 -> Unit Delay/1, Out/1  "VHAL_CANMsgInvalidHRW_flg"

== system halin/HAL_IN/CAN1/VHAL_CANMsgInvalidTC1_flg ==
  Cast To Boolean13 : DataTypeConversion  OutDataTypeStr=boolean
  Constant : Constant  Value=TRUE
  Latch13 : hcu_lib/Basic_Blocks/Latch
  Switch13 : Switch  Criteria=u2 ~= 0
  Unit Delay : UnitDelay  SampleTime=-1  HasFrameUpgradeWarning=on
  UnitConverter : DataTypeConversion  OutDataTypeStr=boolean
  Out : Outport
  wires:
  Constant/1 -> Switch13/3
  Unit Delay/1 -> Cast To Boolean13/1
  Cast To Boolean13/1 -> Switch13/1, Latch13/1
  Switch13/1 -> UnitConverter/1
  Latch13/1 -> Switch13/2
  UnitConverter/1 -> Unit Delay/1, Out/1  "VHAL_CANMsgInvalidTC1_flg"

== system halin/HAL_IN/CAN2/IVI_C100_0 ==
  DT_CAN2_SG_IVI_C100_0 : Inport
  IVIACFanSpdReqCmd : Subsystem
  bus_selector : BusSelector  OutputSignals=CAN2_IVI_ACFanSpdReq_Cmd
  VHAL_IVIACFanSpdReqCmd_enum : Outport
  wires:
  DT_CAN2_SG_IVI_C100_0/1 -> [DT_CAN2_SG_IVI_C100_0]
  [DT_CAN2_SG_IVI_C100_0] -> bus_selector/1
  bus_selector/1 -> IVIACFanSpdReqCmd/1(IVI_ACFanSpdReq_Cmd)  "<CAN2_IVI_ACFanSpdReq_Cmd>"
  IVIACFanSpdReqCmd/1(VHAL_IVIACFanSpdReqCmd_enum) -> VHAL_IVIACFanSpdReqCmd_enum/1

== system halin/HAL_IN/CAN2/VHAL_CANMsgInvalidIVIC1000_flg ==
  Cast To Boolean13 : DataTypeConversion  OutDataTypeStr=boolean
  Constant : Constant  Value=TRUE
  Latch13 : hcu_lib/Basic_Blocks/Latch
  Switch13 : Switch  Criteria=u2 ~= 0
  Unit Delay : UnitDelay  SampleTime=-1  HasFrameUpgradeWarning=on
  UnitConverter : DataTypeConversion  OutDataTypeStr=boolean
  Out : Outport
  wires:
  Constant/1 -> Switch13/3
  Unit Delay/1 -> Cast To Boolean13/1
  Cast To Boolean13/1 -> Switch13/1, Latch13/1
  Switch13/1 -> UnitConverter/1
  Latch13/1 -> Switch13/2
  UnitConverter/1 -> Unit Delay/1, Out/1  "VHAL_CANMsgInvalidIVIC1000_flg"

== system halin/HAL_IN/CAN3/B2TM_Info ==
  DT_CAN3_SG_B2TM_Info : Inport
  B2THVRlySta : Subsystem
  bus_selector : BusSelector  OutputSignals=CAN3_B2THVRlySta
  VHAL_B2THVRlySta_enum : Outport
  wires:
  DT_CAN3_SG_B2TM_Info/1 -> [DT_CAN3_SG_B2TM_Info]
  [DT_CAN3_SG_B2TM_Info] -> bus_selector/1
  bus_selector/1 -> B2THVRlySta/1(B2THVRlySta)  "<CAN3_B2THVRlySta>"
  B2THVRlySta/1(VHAL_B2THVRlySta_enum) -> VHAL_B2THVRlySta_enum/1

== system halin/HAL_IN/CAN3/B2V_BattInfo1 ==
  DT_CAN3_SG_B2V_BattInfo1 : Inport
  B2VBI1BattType : Subsystem
  bus_selector : BusSelector  OutputSignals=CAN3_B2VBI1BattType
  VHAL_B2VBI1BattType_enum : Outport
  wires:
  DT_CAN3_SG_B2V_BattInfo1/1 -> [DT_CAN3_SG_B2V_BattInfo1]
  [DT_CAN3_SG_B2V_BattInfo1] -> bus_selector/1
  bus_selector/1 -> B2VBI1BattType/1(B2VBI1BattType)  "<CAN3_B2VBI1BattType>"
  B2VBI1BattType/1(VHAL_B2VBI1BattType_enum) -> VHAL_B2VBI1BattType_enum/1

== system halin/HAL_IN/CAN3/B2V_CurrentLimit ==
  DT_CAN3_SG_B2V_CurrentLimit : Inport
  B2VAPlsDischgCurr : Subsystem
  B2VAvaPlsChgCurr : Subsystem
  bus_selector : BusSelector  OutputSignals=CAN3_B2VAPlsDischgCurr
  bus_selector1 : BusSelector  OutputSignals=CAN3_B2VAvaPlsChgCurr
  VHAL_B2VAPlsDischgCurr_A : Outport
  VHAL_B2VAvaPlsChgCurr_A : Outport  Port=2
  wires:
  DT_CAN3_SG_B2V_CurrentLimit/1 -> [DT_CAN3_SG_B2V_CurrentLimit]
  [DT_CAN3_SG_B2V_CurrentLimit] -> bus_selector/1
  bus_selector/1 -> B2VAPlsDischgCurr/1(B2VAPlsDischgCurr)  "<CAN3_B2VAPlsDischgCurr>"
  B2VAPlsDischgCurr/1(VHAL_B2VAPlsDischgCurr_A) -> VHAL_B2VAPlsDischgCurr_A/1
  [DT_CAN3_SG_B2V_CurrentLimit] -> bus_selector1/1
  bus_selector1/1 -> B2VAvaPlsChgCurr/1(B2VAvaPlsChgCurr)  "<CAN3_B2VAvaPlsChgCurr>"
  B2VAvaPlsChgCurr/1(VHAL_B2VAvaPlsChgCurr_A) -> VHAL_B2VAvaPlsChgCurr_A/1

== system halin/HAL_IN/CAN3/B2V_Fult1_32960 ==
  DT_CAN3_SG_B2V_Fult1_32960 : Inport
  B2VHVILFault : Subsystem
  bus_selector : BusSelector  OutputSignals=CAN3_B2VHVILFault
  VHAL_B2VHVILFault_flg : Outport
  wires:
  DT_CAN3_SG_B2V_Fult1_32960/1 -> [DT_CAN3_SG_B2V_Fult1_32960]
  [DT_CAN3_SG_B2V_Fult1_32960] -> bus_selector/1
  bus_selector/1 -> B2VHVILFault/1(B2VHVILFault)  "<CAN3_B2VHVILFault>"
  B2VHVILFault/1(VHAL_B2VHVILFault_flg) -> VHAL_B2VHVILFault_flg/1

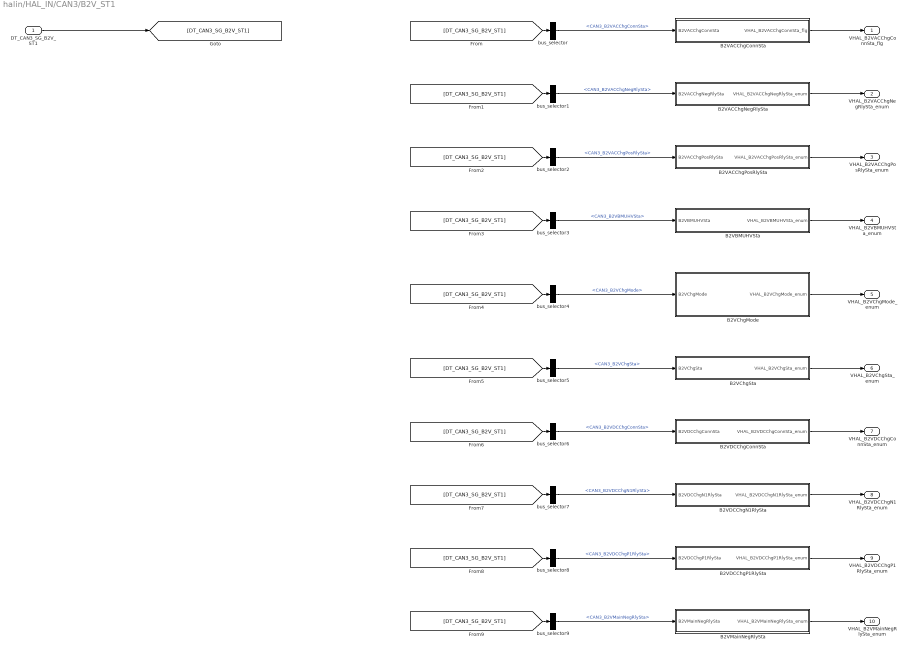
== system halin/HAL_IN/CAN3/B2V_ST1 ==
  DT_CAN3_SG_B2V_ST1 : Inport
  B2VACChgConnSta : Subsystem
  B2VACChgNegRlySta : Subsystem
  B2VACChgPosRlySta : Subsystem
  B2VBMUHVSta : Subsystem
  B2VChgMode : Subsystem
  B2VChgSta : Subsystem
  B2VDCChgConnSta : Subsystem
  B2VDCChgN1RlySta : Subsystem
  B2VDCChgP1RlySta : Subsystem
  B2VMainNegRlySta : Subsystem
  bus_selector : BusSelector  OutputSignals=CAN3_B2VACChgConnSta
  bus_selector1 : BusSelector  OutputSignals=CAN3_B2VACChgNegRlySta
  bus_selector2 : BusSelector  OutputSignals=CAN3_B2VACChgPosRlySta
  bus_selector3 : BusSelector  OutputSignals=CAN3_B2VBMUHVSta
  bus_selector4 : BusSelector  OutputSignals=CAN3_B2VChgMode
  bus_selector5 : BusSelector  OutputSignals=CAN3_B2VChgSta
  bus_selector6 : BusSelector  OutputSignals=CAN3_B2VDCChgConnSta
  bus_selector7 : BusSelector  OutputSignals=CAN3_B2VDCChgN1RlySta
  bus_selector8 : BusSelector  OutputSignals=CAN3_B2VDCChgP1RlySta
  bus_selector9 : BusSelector  OutputSignals=CAN3_B2VMainNegRlySta
  VHAL_B2VACChgConnSta_flg : Outport
  VHAL_B2VACChgNegRlySta_enum : Outport  Port=2
  VHAL_B2VACChgPosRlySta_enum : Outport  Port=3
  VHAL_B2VBMUHVSta_enum : Outport  Port=4
  VHAL_B2VChgMode_enum : Outport  Port=5
  VHAL_B2VChgSta_enum : Outport  Port=6
  VHAL_B2VDCChgConnSta_enum : Outport  Port=7
  VHAL_B2VDCChgN1RlySta_enum : Outport  Port=8
  VHAL_B2VDCChgP1RlySta_enum : Outport  Port=9
  VHAL_B2VMainNegRlySta_enum : Outport  Port=10
  wires:
  DT_CAN3_SG_B2V_ST1/1 -> [DT_CAN3_SG_B2V_ST1]
  [DT_CAN3_SG_B2V_ST1] -> bus_selector/1
  bus_selector/1 -> B2VACChgConnSta/1(B2VACChgConnSta)  "<CAN3_B2VACChgConnSta>"
  B2VACChgConnSta/1(VHAL_B2VACChgConnSta_flg) -> VHAL_B2VACChgConnSta_flg/1
  [DT_CAN3_SG_B2V_ST1] -> bus_selector1/1
  bus_selector1/1 -> B2VACChgNegRlySta/1(B2VACChgNegRlySta)  "<CAN3_B2VACChgNegRlySta>"
  B2VACChgNegRlySta/1(VHAL_B2VACChgNegRlySta_enum) -> VHAL_B2VACChgNegRlySta_enum/1
  [DT_CAN3_SG_B2V_ST1] -> bus_selector2/1
  bus_selector2/1 -> B2VACChgPosRlySta/1(B2VACChgPosRlySta)  "<CAN3_B2VACChgPosRlySta>"
  B2VACChgPosRlySta/1(VHAL_B2VACChgPosRlySta_enum) -> VHAL_B2VACChgPosRlySta_enum/1
  [DT_CAN3_SG_B2V_ST1] -> bus_selector3/1
  bus_selector3/1 -> B2VBMUHVSta/1(B2VBMUHVSta)  "<CAN3_B2VBMUHVSta>"
  B2VBMUHVSta/1(VHAL_B2VBMUHVSta_enum) -> VHAL_B2VBMUHVSta_enum/1
  [DT_CAN3_SG_B2V_ST1] -> bus_selector4/1
  bus_selector4/1 -> B2VChgMode/1(B2VChgMode)  "<CAN3_B2VChgMode>"
  B2VChgMode/1(VHAL_B2VChgMode_enum) -> VHAL_B2VChgMode_enum/1
  [DT_CAN3_SG_B2V_ST1] -> bus_selector5/1
  bus_selector5/1 -> B2VChgSta/1(B2VChgSta)  "<CAN3_B2VChgSta>"
  B2VChgSta/1(VHAL_B2VChgSta_enum) -> VHAL_B2VChgSta_enum/1
  [DT_CAN3_SG_B2V_ST1] -> bus_selector6/1
  bus_selector6/1 -> B2VDCChgConnSta/1(B2VDCChgConnSta)  "<CAN3_B2VDCChgConnSta>"
  B2VDCChgConnSta/1(VHAL_B2VDCChgConnSta_enum) -> VHAL_B2VDCChgConnSta_enum/1
  [DT_CAN3_SG_B2V_ST1] -> bus_selector7/1
  bus_selector7/1 -> B2VDCChgN1RlySta/1(B2VDCChgN1RlySta)  "<CAN3_B2VDCChgN1RlySta>"
  B2VDCChgN1RlySta/1(VHAL_B2VDCChgN1RlySta_enum) -> VHAL_B2VDCChgN1RlySta_enum/1
  [DT_CAN3_SG_B2V_ST1] -> bus_selector8/1
  bus_selector8/1 -> B2VDCChgP1RlySta/1(B2VDCChgP1RlySta)  "<CAN3_B2VDCChgP1RlySta>"
  B2VDCChgP1RlySta/1(VHAL_B2VDCChgP1RlySta_enum) -> VHAL_B2VDCChgP1RlySta_enum/1
  [DT_CAN3_SG_B2V_ST1] -> bus_selector9/1
  bus_selector9/1 -> B2VMainNegRlySta/1(B2VMainNegRlySta)  "<CAN3_B2VMainNegRlySta>"
  B2VMainNegRlySta/1(VHAL_B2VMainNegRlySta_enum) -> VHAL_B2VMainNegRlySta_enum/1

== system halin/HAL_IN/CAN3/B2V_ST2 ==
  DT_CAN3_SG_B2V_ST2 : Inport
  B2VFaultCode : Subsystem
  B2VFaultLv : Subsystem
  B2VPackCurr : Subsystem
  B2VPackInsideVol : Subsystem
  B2VRqHVPwrOff : Subsystem
  B2VSOC : Subsystem
  bus_selector : BusSelector  OutputSignals=CAN3_B2VFaultCode
  bus_selector1 : BusSelector  OutputSignals=CAN3_B2VFaultLv
  bus_selector2 : BusSelector  OutputSignals=CAN3_B2VPackCurr
  bus_selector3 : BusSelector  OutputSignals=CAN3_B2VPackInsideVol
  bus_selector4 : BusSelector  OutputSignals=CAN3_B2VRqHVPwrOff
  bus_selector5 : BusSelector  OutputSignals=CAN3_B2VSOC
  VHAL_B2VFaultCode_enum : Outport
  VHAL_B2VFaultLv_enum : Outport  Port=2
  VHAL_B2VPackCurr_A : Outport  Port=3
  VHAL_B2VPackInsideVol_V : Outport  Port=4
  VHAL_B2VRqHVPwrOff_enum : Outport  Port=5
  VHAL_B2VSOC_pct : Outport  Port=6
  wires:
  DT_CAN3_SG_B2V_ST2/1 -> [DT_CAN3_SG_B2V_ST2]
  [DT_CAN3_SG_B2V_ST2] -> bus_selector/1
  bus_selector/1 -> B2VFaultCode/1(B2VFaultCode)  "<CAN3_B2VFaultCode>"
  B2VFaultCode/1(VHAL_B2VFaultCode_enum) -> VHAL_B2VFaultCode_enum/1
  [DT_CAN3_SG_B2V_ST2] -> bus_selector1/1
  bus_selector1/1 -> B2VFaultLv/1(B2VFaultLv)  "<CAN3_B2VFaultLv>"
  B2VFaultLv/1(VHAL_B2VFaultLv_enum) -> VHAL_B2VFaultLv_enum/1
  [DT_CAN3_SG_B2V_ST2] -> bus_selector2/1
  bus_selector2/1 -> B2VPackCurr/1(B2VPackCurr)  "<CAN3_B2VPackCurr>"
  B2VPackCurr/1(VHAL_B2VPackCurr_A) -> VHAL_B2VPackCurr_A/1
  [DT_CAN3_SG_B2V_ST2] -> bus_selector3/1
  bus_selector3/1 -> B2VPackInsideVol/1(B2VPackInsideVol)  "<CAN3_B2VPackInsideVol>"
  B2VPackInsideVol/1(VHAL_B2VPackInsideVol_V) -> VHAL_B2VPackInsideVol_V/1
  [DT_CAN3_SG_B2V_ST2] -> bus_selector4/1
  bus_selector4/1 -> B2VRqHVPwrOff/1(B2VRqHVPwrOff)  "<CAN3_B2VRqHVPwrOff>"
  B2VRqHVPwrOff/1(VHAL_B2VRqHVPwrOff_enum) -> VHAL_B2VRqHVPwrOff_enum/1
  [DT_CAN3_SG_B2V_ST2] -> bus_selector5/1
  bus_selector5/1 -> B2VSOC/1(B2VSOC)  "<CAN3_B2VSOC>"
  B2VSOC/1(VHAL_B2VSOC_pct) -> VHAL_B2VSOC_pct/1

== system halin/HAL_IN/CAN3/B2V_ST4 ==
  DT_CAN3_SG_B2V_ST4 : Inport
  B2VMinTempPos : Subsystem
  bus_selector : BusSelector  OutputSignals=CAN3_B2VMinTempPos
  VHAL_B2VMinTempPos_enum : Outport
  wires:
  DT_CAN3_SG_B2V_ST4/1 -> [DT_CAN3_SG_B2V_ST4]
  [DT_CAN3_SG_B2V_ST4] -> bus_selector/1
  bus_selector/1 -> B2VMinTempPos/1(B2VMinTempPos)  "<CAN3_B2VMinTempPos>"
  B2VMinTempPos/1(VHAL_B2VMinTempPos_enum) -> VHAL_B2VMinTempPos_enum/1

== system halin/HAL_IN/CAN3/B2V_ST5 ==
  DT_CAN3_SG_B2V_ST5 : Inport
  B2VCellMinVol : Subsystem
  bus_selector : BusSelector  OutputSignals=CAN3_B2VCellMinVol
  VHAL_B2VCellMinVol_V : Outport
  wires:
  DT_CAN3_SG_B2V_ST5/1 -> [DT_CAN3_SG_B2V_ST5]
  [DT_CAN3_SG_B2V_ST5] -> bus_selector/1
  bus_selector/1 -> B2VCellMinVol/1(B2VCellMinVol)  "<CAN3_B2VCellMinVol>"
  B2VCellMinVol/1(VHAL_B2VCellMinVol_V) -> VHAL_B2VCellMinVol_V/1

== system halin/HAL_IN/CAN3/EWP1 ==
  DT_CAN3_SG_EWP1 : Inport
  EWPPEFault : Subsystem
  bus_selector : BusSelector  OutputSignals=CAN3_EWPPEFault
  VHAL_EWPPEFault_enum : Outport
  wires:
  DT_CAN3_SG_EWP1/1 -> [DT_CAN3_SG_EWP1]
  [DT_CAN3_SG_EWP1] -> bus_selector/1
  bus_selector/1 -> EWPPEFault/1(EWPPEFault)  "<CAN3_EWPPEFault>"
  EWPPEFault/1(VHAL_EWPPEFault_enum) -> VHAL_EWPPEFault_enum/1

== system halin/HAL_IN/CAN3/TM_MCUSta1 ==
  DT_CAN3_SG_TM_MCUSta1 : Inport
  AtvDisChgEnFbk : Subsystem
  MCUCtrlMdSta : Subsystem
  MCUIGBTEnFbk : Subsystem
  MotorSpd : Subsystem
  MotorTrq : Subsystem
  bus_selector : BusSelector  OutputSignals=CAN3_AtvDisChgEnFbk
  bus_selector1 : BusSelector  OutputSignals=CAN3_MCUCtrlMdSta
  bus_selector2 : BusSelector  OutputSignals=CAN3_MCUIGBTEnFbk
  bus_selector3 : BusSelector  OutputSignals=CAN3_MotorSpd
  bus_selector4 : BusSelector  OutputSignals=CAN3_MotorTrq
  VHAL_AtvDisChgEnFbk_flg : Outport
  VHAL_MCUCtrlMdSta_enum : Outport  Port=2
  VHAL_MCUIGBTEnFbk_flg : Outport  Port=3
  VHAL_MotorSpd_rpm : Outport  Port=4
  VHAL_MotorTrq_Nm : Outport  Port=5
  wires:
  DT_CAN3_SG_TM_MCUSta1/1 -> [DT_CAN3_SG_TM_MCUSta1]
  [DT_CAN3_SG_TM_MCUSta1] -> bus_selector/1
  bus_selector/1 -> AtvDisChgEnFbk/1(AtvDisChgEnFbk)  "<CAN3_AtvDisChgEnFbk>"
  AtvDisChgEnFbk/1(VHAL_AtvDisChgEnFbk_flg) -> VHAL_AtvDisChgEnFbk_flg/1
  [DT_CAN3_SG_TM_MCUSta1] -> bus_selector1/1
  bus_selector1/1 -> MCUCtrlMdSta/1(MCUCtrlMdSta)  "<CAN3_MCUCtrlMdSta>"
  MCUCtrlMdSta/1(VHAL_MCUCtrlMdSta_enum) -> VHAL_MCUCtrlMdSta_enum/1
  [DT_CAN3_SG_TM_MCUSta1] -> bus_selector2/1
  bus_selector2/1 -> MCUIGBTEnFbk/1(MCUIGBTEnFbk)  "<CAN3_MCUIGBTEnFbk>"
  MCUIGBTEnFbk/1(VHAL_MCUIGBTEnFbk_flg) -> VHAL_MCUIGBTEnFbk_flg/1
  [DT_CAN3_SG_TM_MCUSta1] -> bus_selector3/1
  bus_selector3/1 -> MotorSpd/1(MotorSpd)  "<CAN3_MotorSpd>"
  MotorSpd/1(VHAL_MotorSpd_rpm) -> VHAL_MotorSpd_rpm/1
  [DT_CAN3_SG_TM_MCUSta1] -> bus_selector4/1
  bus_selector4/1 -> MotorTrq/1(MotorTrq)  "<CAN3_MotorTrq>"
  MotorTrq/1(VHAL_MotorTrq_Nm) -> VHAL_MotorTrq_Nm/1

== system halin/HAL_IN/CAN3/TM_MCUSta2 ==
  DT_CAN3_SG_TM_MCUSta2 : Inport
  MCUFailGrade : Subsystem
  MCUTemp : Subsystem
  MCUTrqLimHi : Subsystem
  MCUTrqLimLo : Subsystem
  MotorTemp : Subsystem
  bus_selector : BusSelector  OutputSignals=CAN3_MCUFailGrade
  bus_selector1 : BusSelector  OutputSignals=CAN3_MCUTemp
  bus_selector2 : BusSelector  OutputSignals=CAN3_MCUTrqLimHi
  bus_selector3 : BusSelector  OutputSignals=CAN3_MCUTrqLimLo
  bus_selector4 : BusSelector  OutputSignals=CAN3_MotorTemp
  VHAL_MCUFailGrade_enum : Outport
  VHAL_MCUTemp_C : Outport  Port=2
  VHAL_MCUTrqLimHi_Nm : Outport  Port=3
  VHAL_MCUTrqLimLo_Nm : Outport  Port=4
  VHAL_MotorTemp_C : Outport  Port=5
  wires:
  DT_CAN3_SG_TM_MCUSta2/1 -> [DT_CAN3_SG_TM_MCUSta2]
  [DT_CAN3_SG_TM_MCUSta2] -> bus_selector/1
  bus_selector/1 -> MCUFailGrade/1(MCUFailGrade)  "<CAN3_MCUFailGrade>"
  MCUFailGrade/1(VHAL_MCUFailGrade_enum) -> VHAL_MCUFailGrade_enum/1
  [DT_CAN3_SG_TM_MCUSta2] -> bus_selector1/1
  bus_selector1/1 -> MCUTemp/1(MCUTemp)  "<CAN3_MCUTemp>"
  MCUTemp/1(VHAL_MCUTemp_C) -> VHAL_MCUTemp_C/1
  [DT_CAN3_SG_TM_MCUSta2] -> bus_selector2/1
  bus_selector2/1 -> MCUTrqLimHi/1(MCUTrqLimHi)  "<CAN3_MCUTrqLimHi>"
  MCUTrqLimHi/1(VHAL_MCUTrqLimHi_Nm) -> VHAL_MCUTrqLimHi_Nm/1
  [DT_CAN3_SG_TM_MCUSta2] -> bus_selector3/1
  bus_selector3/1 -> MCUTrqLimLo/1(MCUTrqLimLo)  "<CAN3_MCUTrqLimLo>"
  MCUTrqLimLo/1(VHAL_MCUTrqLimLo_Nm) -> VHAL_MCUTrqLimLo_Nm/1
  [DT_CAN3_SG_TM_MCUSta2] -> bus_selector4/1
  bus_selector4/1 -> MotorTemp/1(MotorTemp)  "<CAN3_MotorTemp>"
  MotorTemp/1(VHAL_MotorTemp_C) -> VHAL_MotorTemp_C/1

== system halin/HAL_IN/CAN3/TM_MCUSta3 ==
  DT_CAN3_SG_TM_MCUSta3 : Inport
  MCUDCCur : Subsystem
  MCUDCVol : Subsystem
  MCUFailCode : Subsystem
  bus_selector : BusSelector  OutputSignals=CAN3_MCUDCCur
  bus_selector1 : BusSelector  OutputSignals=CAN3_MCUDCVol
  bus_selector2 : BusSelector  OutputSignals=CAN3_MCUFailCode
  VHAL_MCUDCCur_A : Outport
  VHAL_MCUDCVol_V : Outport  Port=2
  VHAL_MCUFailCode_enum : Outport  Port=3
  wires:
  DT_CAN3_SG_TM_MCUSta3/1 -> [DT_CAN3_SG_TM_MCUSta3]
  [DT_CAN3_SG_TM_MCUSta3] -> bus_selector/1
  bus_selector/1 -> MCUDCCur/1(MCUDCCur)  "<CAN3_MCUDCCur>"
  MCUDCCur/1(VHAL_MCUDCCur_A) -> VHAL_MCUDCCur_A/1
  [DT_CAN3_SG_TM_MCUSta3] -> bus_selector1/1
  bus_selector1/1 -> MCUDCVol/1(MCUDCVol)  "<CAN3_MCUDCVol>"
  MCUDCVol/1(VHAL_MCUDCVol_V) -> VHAL_MCUDCVol_V/1
  [DT_CAN3_SG_TM_MCUSta3] -> bus_selector2/1
  bus_selector2/1 -> MCUFailCode/1(MCUFailCode)  "<CAN3_MCUFailCode>"
  MCUFailCode/1(VHAL_MCUFailCode_enum) -> VHAL_MCUFailCode_enum/1

== system halin/HAL_IN/CAN3/VHAL_CANMsgInvalidB2TMInfo_flg ==
  Cast To Boolean13 : DataTypeConversion  OutDataTypeStr=boolean
  Constant : Constant  Value=TRUE
  Latch13 : hcu_lib/Basic_Blocks/Latch
  Switch13 : Switch  Criteria=u2 ~= 0
  Unit Delay : UnitDelay  SampleTime=-1  HasFrameUpgradeWarning=on
  UnitConverter : DataTypeConversion  OutDataTypeStr=boolean
  Out : Outport
  wires:
  Constant/1 -> Switch13/3
  Unit Delay/1 -> Cast To Boolean13/1
  Cast To Boolean13/1 -> Switch13/1, Latch13/1
  Switch13/1 -> UnitConverter/1
  Latch13/1 -> Switch13/2
  UnitConverter/1 -> Unit Delay/1, Out/1  "VHAL_CANMsgInvalidB2TMInfo_flg"

== system halin/HAL_IN/CAN3/VHAL_CANMsgInvalidB2VBattInfo1_flg ==
  Cast To Boolean13 : DataTypeConversion  OutDataTypeStr=boolean
  Constant : Constant  Value=TRUE
  Latch13 : hcu_lib/Basic_Blocks/Latch
  Switch13 : Switch  Criteria=u2 ~= 0
  Unit Delay : UnitDelay  SampleTime=-1  HasFrameUpgradeWarning=on
  UnitConverter : DataTypeConversion  OutDataTypeStr=boolean
  Out : Outport
  wires:
  Constant/1 -> Switch13/3
  Unit Delay/1 -> Cast To Boolean13/1
  Cast To Boolean13/1 -> Switch13/1, Latch13/1
  Switch13/1 -> UnitConverter/1
  Latch13/1 -> Switch13/2
  UnitConverter/1 -> Unit Delay/1, Out/1  "VHAL_CANMsgInvalidB2VBattInfo1_flg"

== system halin/HAL_IN/CAN3/VHAL_CANMsgInvalidB2VCurrentLimit_flg ==
  Cast To Boolean13 : DataTypeConversion  OutDataTypeStr=boolean
  Constant : Constant  Value=TRUE
  Latch13 : hcu_lib/Basic_Blocks/Latch
  Switch13 : Switch  Criteria=u2 ~= 0
  Unit Delay : UnitDelay  SampleTime=-1  HasFrameUpgradeWarning=on
  UnitConverter : DataTypeConversion  OutDataTypeStr=boolean
  Out : Outport
  wires:
  Constant/1 -> Switch13/3
  Unit Delay/1 -> Cast To Boolean13/1
  Cast To Boolean13/1 -> Switch13/1, Latch13/1
  Switch13/1 -> UnitConverter/1
  Latch13/1 -> Switch13/2
  UnitConverter/1 -> Unit Delay/1, Out/1  "VHAL_CANMsgInvalidB2VCurrentLimit_flg"

== system halin/HAL_IN/CAN3/VHAL_CANMsgInvalidB2VFult132960_flg ==
  Cast To Boolean13 : DataTypeConversion  OutDataTypeStr=boolean
  Constant : Constant  Value=TRUE
  Latch13 : hcu_lib/Basic_Blocks/Latch
  Switch13 : Switch  Criteria=u2 ~= 0
  Unit Delay : UnitDelay  SampleTime=-1  HasFrameUpgradeWarning=on
  UnitConverter : DataTypeConversion  OutDataTypeStr=boolean
  Out : Outport
  wires:
  Constant/1 -> Switch13/3
  Unit Delay/1 -> Cast To Boolean13/1
  Cast To Boolean13/1 -> Switch13/1, Latch13/1
  Switch13/1 -> UnitConverter/1
  Latch13/1 -> Switch13/2
  UnitConverter/1 -> Unit Delay/1, Out/1  "VHAL_CANMsgInvalidB2VFult132960_flg"

== system halin/HAL_IN/CAN3/VHAL_CANMsgInvalidB2VST1_flg ==
  Cast To Boolean13 : DataTypeConversion  OutDataTypeStr=boolean
  Constant : Constant  Value=TRUE
  Latch13 : hcu_lib/Basic_Blocks/Latch
  Switch13 : Switch  Criteria=u2 ~= 0
  Unit Delay : UnitDelay  SampleTime=-1  HasFrameUpgradeWarning=on
  UnitConverter : DataTypeConversion  OutDataTypeStr=boolean
  Out : Outport
  wires:
  Constant/1 -> Switch13/3
  Unit Delay/1 -> Cast To Boolean13/1
  Cast To Boolean13/1 -> Switch13/1, Latch13/1
  Switch13/1 -> UnitConverter/1
  Latch13/1 -> Switch13/2
  UnitConverter/1 -> Unit Delay/1, Out/1  "VHAL_CANMsgInvalidB2VST1_flg"

== system halin/HAL_IN/CAN3/VHAL_CANMsgInvalidB2VST2_flg ==
  Cast To Boolean13 : DataTypeConversion  OutDataTypeStr=boolean
  Constant : Constant  Value=TRUE
  Latch13 : hcu_lib/Basic_Blocks/Latch
  Switch13 : Switch  Criteria=u2 ~= 0
  Unit Delay : UnitDelay  SampleTime=-1  HasFrameUpgradeWarning=on
  UnitConverter : DataTypeConversion  OutDataTypeStr=boolean
  Out : Outport
  wires:
  Constant/1 -> Switch13/3
  Unit Delay/1 -> Cast To Boolean13/1
  Cast To Boolean13/1 -> Switch13/1, Latch13/1
  Switch13/1 -> UnitConverter/1
  Latch13/1 -> Switch13/2
  UnitConverter/1 -> Unit Delay/1, Out/1  "VHAL_CANMsgInvalidB2VST2_flg"

== system halin/HAL_IN/CAN3/VHAL_CANMsgInvalidB2VST4_flg ==
  Cast To Boolean13 : DataTypeConversion  OutDataTypeStr=boolean
  Constant : Constant  Value=TRUE
  Latch13 : hcu_lib/Basic_Blocks/Latch
  Switch13 : Switch  Criteria=u2 ~= 0
  Unit Delay : UnitDelay  SampleTime=-1  HasFrameUpgradeWarning=on
  UnitConverter : DataTypeConversion  OutDataTypeStr=boolean
  Out : Outport
  wires:
  Constant/1 -> Switch13/3
  Unit Delay/1 -> Cast To Boolean13/1
  Cast To Boolean13/1 -> Switch13/1, Latch13/1
  Switch13/1 -> UnitConverter/1
  Latch13/1 -> Switch13/2
  UnitConverter/1 -> Unit Delay/1, Out/1  "VHAL_CANMsgInvalidB2VST4_flg"

== system halin/HAL_IN/CAN3/VHAL_CANMsgInvalidB2VST5_flg ==
  Cast To Boolean13 : DataTypeConversion  OutDataTypeStr=boolean
  Constant : Constant  Value=TRUE
  Latch13 : hcu_lib/Basic_Blocks/Latch
  Switch13 : Switch  Criteria=u2 ~= 0
  Unit Delay : UnitDelay  SampleTime=-1  HasFrameUpgradeWarning=on
  UnitConverter : DataTypeConversion  OutDataTypeStr=boolean
  Out : Outport
  wires:
  Constant/1 -> Switch13/3
  Unit Delay/1 -> Cast To Boolean13/1
  Cast To Boolean13/1 -> Switch13/1, Latch13/1
  Switch13/1 -> UnitConverter/1
  Latch13/1 -> Switch13/2
  UnitConverter/1 -> Unit Delay/1, Out/1  "VHAL_CANMsgInvalidB2VST5_flg"

== system halin/HAL_IN/CAN3/VHAL_CANMsgInvalidEWP1_flg ==
  Cast To Boolean13 : DataTypeConversion  OutDataTypeStr=boolean
  Constant : Constant  Value=TRUE
  Latch13 : hcu_lib/Basic_Blocks/Latch
  Switch13 : Switch  Criteria=u2 ~= 0
  Unit Delay : UnitDelay  SampleTime=-1  HasFrameUpgradeWarning=on
  UnitConverter : DataTypeConversion  OutDataTypeStr=boolean
  Out : Outport
  wires:
  Constant/1 -> Switch13/3
  Unit Delay/1 -> Cast To Boolean13/1
  Cast To Boolean13/1 -> Switch13/1, Latch13/1
  Switch13/1 -> UnitConverter/1
  Latch13/1 -> Switch13/2
  UnitConverter/1 -> Unit Delay/1, Out/1  "VHAL_CANMsgInvalidEWP1_flg"

== system halin/HAL_IN/CAN3/VHAL_CANMsgInvalidTMMCUSta1_flg ==
  Cast To Boolean13 : DataTypeConversion  OutDataTypeStr=boolean
  Constant : Constant  Value=TRUE
  Latch13 : hcu_lib/Basic_Blocks/Latch
  Switch13 : Switch  Criteria=u2 ~= 0
  Unit Delay : UnitDelay  SampleTime=-1  HasFrameUpgradeWarning=on
  UnitConverter : DataTypeConversion  OutDataTypeStr=boolean
  Out : Outport
  wires:
  Constant/1 -> Switch13/3
  Unit Delay/1 -> Cast To Boolean13/1
  Cast To Boolean13/1 -> Switch13/1, Latch13/1
  Switch13/1 -> UnitConverter/1
  Latch13/1 -> Switch13/2
  UnitConverter/1 -> Unit Delay/1, Out/1  "VHAL_CANMsgInvalidTMMCUSta1_flg"

== system halin/HAL_IN/CAN3/VHAL_CANMsgInvalidTMMCUSta2_flg ==
  Cast To Boolean13 : DataTypeConversion  OutDataTypeStr=boolean
  Constant : Constant  Value=TRUE
  Latch13 : hcu_lib/Basic_Blocks/Latch
  Switch13 : Switch  Criteria=u2 ~= 0
  Unit Delay : UnitDelay  SampleTime=-1  HasFrameUpgradeWarning=on
  UnitConverter : DataTypeConversion  OutDataTypeStr=boolean
  Out : Outport
  wires:
  Constant/1 -> Switch13/3
  Unit Delay/1 -> Cast To Boolean13/1
  Cast To Boolean13/1 -> Switch13/1, Latch13/1
  Switch13/1 -> UnitConverter/1
  Latch13/1 -> Switch13/2
  UnitConverter/1 -> Unit Delay/1, Out/1  "VHAL_CANMsgInvalidTMMCUSta2_flg"

== system halin/HAL_IN/CAN3/VHAL_CANMsgInvalidTMMCUSta3_flg ==
  Cast To Boolean13 : DataTypeConversion  OutDataTypeStr=boolean
  Constant : Constant  Value=TRUE
  Latch13 : hcu_lib/Basic_Blocks/Latch
  Switch13 : Switch  Criteria=u2 ~= 0
  Unit Delay : UnitDelay  SampleTime=-1  HasFrameUpgradeWarning=on
  UnitConverter : DataTypeConversion  OutDataTypeStr=boolean
  Out : Outport
  wires:
  Constant/1 -> Switch13/3
  Unit Delay/1 -> Cast To Boolean13/1
  Cast To Boolean13/1 -> Switch13/1, Latch13/1
  Switch13/1 -> UnitConverter/1
  Latch13/1 -> Switch13/2
  UnitConverter/1 -> Unit Delay/1, Out/1  "VHAL_CANMsgInvalidTMMCUSta3_flg"

== system halin/HAL_IN/CAN4/VHAL_CANMsgInvalidZFRC1000_flg ==
  Cast To Boolean13 : DataTypeConversion  OutDataTypeStr=boolean
  Constant : Constant  Value=TRUE
  Latch13 : hcu_lib/Basic_Blocks/Latch
  Switch13 : Switch  Criteria=u2 ~= 0
  Unit Delay : UnitDelay  SampleTime=-1  HasFrameUpgradeWarning=on
  UnitConverter : DataTypeConversion  OutDataTypeStr=boolean
  Out : Outport
  wires:
  Constant/1 -> Switch13/3
  Unit Delay/1 -> Cast To Boolean13/1
  Cast To Boolean13/1 -> Switch13/1, Latch13/1
  Switch13/1 -> UnitConverter/1
  Latch13/1 -> Switch13/2
  UnitConverter/1 -> Unit Delay/1, Out/1  "VHAL_CANMsgInvalidZFRC1000_flg"

== system halin/HAL_IN/CAN4/VHAL_CANMsgInvalidZFRCE1000_flg ==
  Cast To Boolean13 : DataTypeConversion  OutDataTypeStr=boolean
  Constant : Constant  Value=TRUE
  Latch13 : hcu_lib/Basic_Blocks/Latch
  Switch13 : Switch  Criteria=u2 ~= 0
  Unit Delay : UnitDelay  SampleTime=-1  HasFrameUpgradeWarning=on
  UnitConverter : DataTypeConversion  OutDataTypeStr=boolean
  Out : Outport
  wires:
  Constant/1 -> Switch13/3
  Unit Delay/1 -> Cast To Boolean13/1
  Cast To Boolean13/1 -> Switch13/1, Latch13/1
  Switch13/1 -> UnitConverter/1
  Latch13/1 -> Switch13/2
  UnitConverter/1 -> Unit Delay/1, Out/1  "VHAL_CANMsgInvalidZFRCE1000_flg"

== system halin/HAL_IN/CAN4/VHAL_CANMsgInvalidZRRCE1000_flg ==
  Cast To Boolean13 : DataTypeConversion  OutDataTypeStr=boolean
  Constant : Constant  Value=TRUE
  Latch13 : hcu_lib/Basic_Blocks/Latch
  Switch13 : Switch  Criteria=u2 ~= 0
  Unit Delay : UnitDelay  SampleTime=-1  HasFrameUpgradeWarning=on
  UnitConverter : DataTypeConversion  OutDataTypeStr=boolean
  Out : Outport
  wires:
  Constant/1 -> Switch13/3
  Unit Delay/1 -> Cast To Boolean13/1
  Cast To Boolean13/1 -> Switch13/1, Latch13/1
  Switch13/1 -> UnitConverter/1
  Latch13/1 -> Switch13/2
  UnitConverter/1 -> Unit Delay/1, Out/1  "VHAL_CANMsgInvalidZRRCE1000_flg"

== system halin/HAL_IN/CAN4/VHAL_CANMsgInvalidZRRCE1001_flg ==
  Cast To Boolean13 : DataTypeConversion  OutDataTypeStr=boolean
  Constant : Constant  Value=TRUE
  Latch13 : hcu_lib/Basic_Blocks/Latch
  Switch13 : Switch  Criteria=u2 ~= 0
  Unit Delay : UnitDelay  SampleTime=-1  HasFrameUpgradeWarning=on
  UnitConverter : DataTypeConversion  OutDataTypeStr=boolean
  Out : Outport
  wires:
  Constant/1 -> Switch13/3
  Unit Delay/1 -> Cast To Boolean13/1
  Cast To Boolean13/1 -> Switch13/1, Latch13/1
  Switch13/1 -> UnitConverter/1
  Latch13/1 -> Switch13/2
  UnitConverter/1 -> Unit Delay/1, Out/1  "VHAL_CANMsgInvalidZRRCE1001_flg"

== system halin/HAL_IN/CAN4/VHAL_CANMsgInvalidzGWCANRr1C500_flg ==
  Cast To Boolean13 : DataTypeConversion  OutDataTypeStr=boolean
  Constant : Constant  Value=TRUE
  Latch13 : hcu_lib/Basic_Blocks/Latch
  Switch13 : Switch  Criteria=u2 ~= 0
  Unit Delay : UnitDelay  SampleTime=-1  HasFrameUpgradeWarning=on
  UnitConverter : DataTypeConversion  OutDataTypeStr=boolean
  Out : Outport
  wires:
  Constant/1 -> Switch13/3
  Unit Delay/1 -> Cast To Boolean13/1
  Cast To Boolean13/1 -> Switch13/1, Latch13/1
  Switch13/1 -> UnitConverter/1
  Latch13/1 -> Switch13/2
  UnitConverter/1 -> Unit Delay/1, Out/1  "VHAL_CANMsgInvalidzGWCANRr1C500_flg"

== system halin/HAL_IN/CAN4/ZFR_C100_0 ==
  DT_CAN4_SG_ZFR_C100_0 : Inport
  ParkBrakeSW : Subsystem
  bus_selector : BusSelector  OutputSignals=CAN4_ParkBrakeSW
  VHAL_ParkBrakeSW_enum : Outport
  wires:
  DT_CAN4_SG_ZFR_C100_0/1 -> [DT_CAN4_SG_ZFR_C100_0]
  [DT_CAN4_SG_ZFR_C100_0] -> bus_selector/1
  bus_selector/1 -> ParkBrakeSW/1(ParkBrakeSW)  "<CAN4_ParkBrakeSW>"
  ParkBrakeSW/1(VHAL_ParkBrakeSW_enum) -> VHAL_ParkBrakeSW_enum/1
